simulink model "Systems_Analysis_with_Disturbance"  (R2023a)
settings: Solver=VariableStepAuto  StartTime=0.0  StopTime=10.0  RelTol=1e-3
settings Model: Creator=Mohamed Ezzelrgal  LastModifiedBy=Mohamed Ezzelrgal

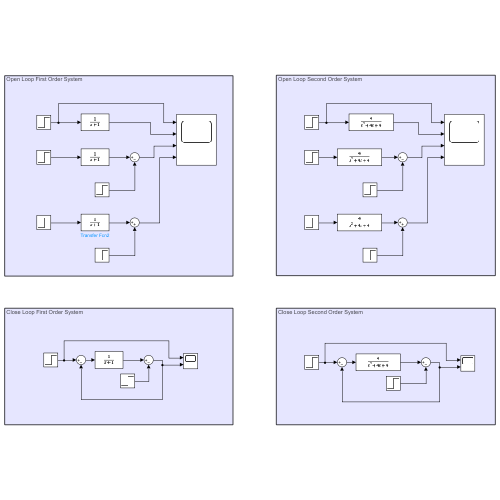
[thumbnail: Simulink's stored preview of the top-level diagram]
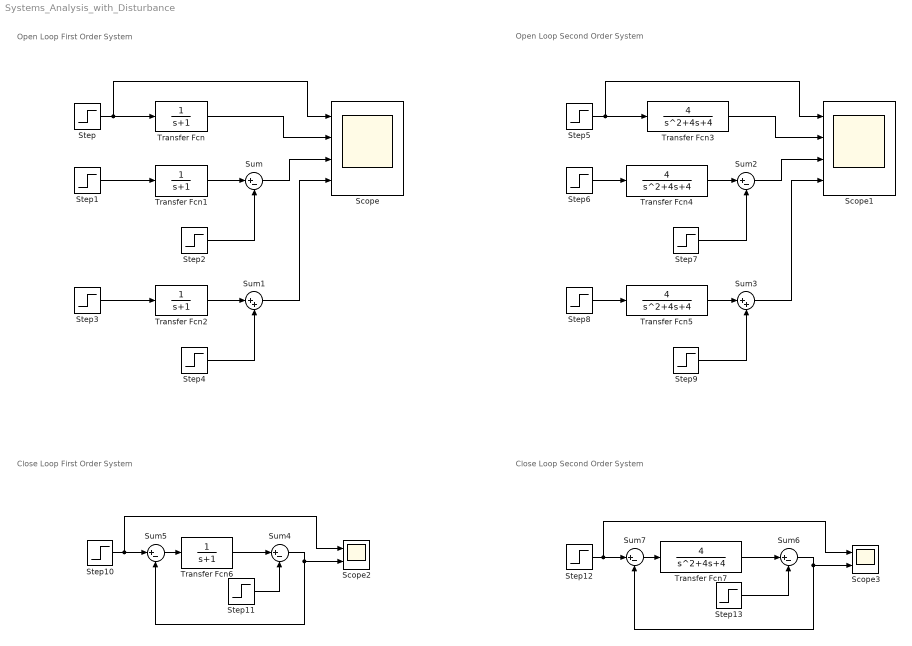
== system Systems_Analysis_with_Disturbance ==
  note: Close Loop Second Order System
  note: Close Loop First Order System
  note: Open Loop Second Order System
  note: Open Loop First Order System
  Scope : Scope  NumInputPorts=4
  Scope1 : Scope  NumInputPorts=4
  Scope2 : Scope  NumInputPorts=2
  Scope3 : Scope  NumInputPorts=2
  Step{,1,3,5..6,8,10,12} (8 alike) : Step  SampleTime=0
  Step11 : Step  Time=5  After=0.3  SampleTime=0
  Step13 : Step  Time=3  After=1.2  SampleTime=0
  Step{2,4,7,9} (4 alike) : Step  Time=3  After=0.7  SampleTime=0
  Sum{,2,4..7} (6 alike) : Sum  Inputs=|+-
  Sum1 : Sum  Inputs=|++
  Sum3 : Sum  Inputs=|++
  Transfer Fcn{,1..2,6} (4 alike) : TransferFcn  Denominator=[1 1]
  Transfer Fcn{3..5,7} (4 alike) : TransferFcn  Numerator=[4]  Denominator=[1 4 4]
  wires:
  Step/1 -> Scope/1, Transfer Fcn/1
  Transfer Fcn/1 -> Scope/2
  Step1/1 -> Transfer Fcn1/1
  Transfer Fcn1/1 -> Sum/1
  Step2/1 -> Sum/2
  Sum/1 -> Scope/3
  Sum1/1 -> Scope/4
  Step4/1 -> Sum1/2
  Transfer Fcn2/1 -> Sum1/1
  Step3/1 -> Transfer Fcn2/1
  Step9/1 -> Sum3/2
  Sum3/1 -> Scope1/4
  Sum2/1 -> Scope1/3
  Step7/1 -> Sum2/2
  Transfer Fcn3/1 -> Scope1/2
  Step5/1 -> Transfer Fcn3/1, Scope1/1
  Step6/1 -> Transfer Fcn4/1
  Transfer Fcn4/1 -> Sum2/1
  Transfer Fcn5/1 -> Sum3/1
  Step8/1 -> Transfer Fcn5/1
  Transfer Fcn6/1 -> Sum4/1
  Step11/1 -> Sum4/2
  Sum5/1 -> Transfer Fcn6/1
  Step10/1 -> Scope2/1, Sum5/1
  Sum4/1 -> Scope2/2, Sum5/2
  Sum6/1 -> Sum7/2, Scope3/2
  Step12/1 -> Sum7/1, Scope3/1
  Sum7/1 -> Transfer Fcn7/1
  Step13/1 -> Sum6/2
  Transfer Fcn7/1 -> Sum6/1
